simulink model "rpoco8_100_r2"  (R2013a)
settings: Solver=VariableStepDiscrete  SolverMode=SingleTasking  StartTime=0.0  StopTime=10.0  RelTol=1e-3
libraries: xbsIndex_r4 x2263, casper_library_misc x52, casper_library_multipliers x19, xps_library x5, casper_library_sources x4, casper_library_delays x1
(part 1 of 27)
settings Model: Creator=mdexter  LastModifiedBy=domagalski
settings DataIOCC: SignalLoggingSaveFormat=ModelDataLogs
settings OptimizationCC: InlineParams=on  ExpressionDepthLimit=2147483647
settings DebuggingCC: FcnCallInpInsideContextMsg=EnableAllAsWarning

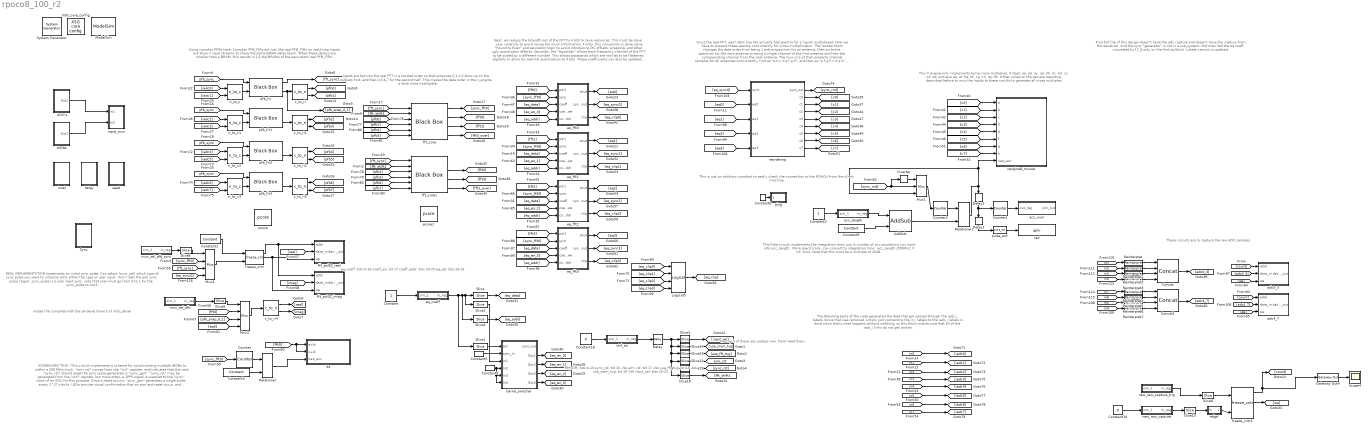
== system rpoco8_100_r2 ==
  note: model file compiled with the s6-devel branch of mlib_devel
  note: !DISREGARD THIS !
      |
      | This circuit implements a scheme for synchronizing
      | multiple IBOBs to within a 200 MHz clock.  "arm_rst"
      | comes from the "ctrl" register, and indicates that the
      | next "sync_rst" should reset the sync pulse generated
      | in "sync_gen".  "sync_rst" may be generated from
      | the "ctrl" register, but more often, a 1PPS signal is
      | supplied to the "sync" input of an ADC for this
      | purpose.  Once a reset occurs, "sync_gen" generates
      | a single pulse every 2^27 clocks.  LEDs provide visual
      | confirmation that an arm and reset occur, and "mrst"
      | is passed over XAUI for the purpose of informing
      | downstream logic in a packetized correlator that
      | a "master reset" has occurred.
  note: Next, we reduce the bitwidth out of the FFT to 4 bits to save resources.
      | This must be done very carefully to avoid losing too much information.
      | Firstly, this conversion is done using "Round to Even" and saturation
      | logic to avoid introducing DC offsets, wrapping, and other ugly quantizaton
      | effects.  Secondly, the "equalizer" allows each frequency channel of the
      | FFT to be scaled by a different number.  This allows passbands which are
      | not flat to be flattened digitally to allow for optimal quantization to 4 bits.
      | These coefficients can also be updated dynamically for gain control.
      | Coefficients can be dynamically written into the "equalizer" by
      | specifying the channel ("coeff_addr") and the value of the
      | coefficient ("coeff"), and then using "coeff_en" to write the
      | new coefficient into the equalization table.
  note: eq_coeff: bits 0-16
      | coeff_en: bit 17
      | coeff_addr: bits 20-25
      | eq_sel: bits 28-31
  note: fft_shift: bits 0-15
      | sync_rst: bit 16 -NA
      | arm_rst: bit 17 -NA
      | use_fft_tvg: bit 18 -NA
      | use_sram_tvg: bit 19 -NA
      | input_sel: bits 20-22
  note: Since the real-FFT, each data line has actually had spectra for 2 inputs multiplexed.
      | Now we have to present these spectra concurrently for cross-multiplication.  The reorder
      | block changes the data order from being 1 entire spectrum for an antenna, then an entire
      | spectrum for the next antenna to being a single channel of the first antenna and then the
      | corresponding channel from the next antenna.  The mux circuit then presents channel
      | samples for all antennas concurrently, first as "a b c d e f g h", and then as "e f g h c d a b".
      | We can post samples twice b/c for 8 data lines, data is only valid 1/2 the time.  By posting
      | samples twice with permuted order, we can cut out some cmults in the xengine that follows.
  note: This X engine only implements some cross-multiplies.  It does:
      | aa, ab, ac, ad, bb, bc, bd, cc, cd, dd, and also
      | ae, af, be, bf, cg, ch, dg, dh.  It then relies on the sample
      | reposting described before to mux the inputs to these
      | cmults to generate all cross multiples.
  note: Inputs are fed into the real FFT in a twisted order
      | so that antennas 0,1,2,3 show up on the outputs first,
      | and then 4,5,6,7 for the second half.  This makes the
      | data order in the x_engine a little more intelligible.
  note: Using complex PFBs here.  Complex PFB_FIRs act just like real
      | PFB_FIRs on real/imag inputs, but  allow 2 input streams to
      | share the same BRAM delay block.  When these delays are smaller
      | than a BRAM, this results in 1/2 the BRAMs of the equivalent real
      | PFB_FIRs.
  note: the top 5 of these are
      | useless now. Dont
      | need them.
  note: REAL IMPLEMENTATION
      |
      | Impements an initial sync pulse.
      | Can select (sync_sel) which type of
      | sync pulse you want to initialize with; either the
      | 1pps or  user input.
      | "Arm"  sets the adc sync pulse (1pps).
      | sync_pulse is a user  input sync. note that
      | user must go from 0 to 1 for the sync_pulse to
      | work.
  note: This little circuit implements the integration time.
      | put in number of accumulations you want into acc_length..
      | More specifically,  can convert to integration time : acc_length /200MHz = int. time.
      | Note that  this must be a multiple of 2048.
  note: These circuits are to capture the raw ADC samples.
  note: First bof file of this design doesn't have the adc
      | capture and doesn't have the capture from the
      | equalizer. And the sync "generator" is not in a sub_system.
      | Old ones had the  eq coeff converted to 17_6 only on the
      | first eq block.
      | Latest version is updated.
  note: The Walshing parts of the code generated the data
      | that got passed through the iadc_i labels. Since that
      | was removed, simply just connecting the in_i labels to
      | the iadc_i labels is done since that's what happens
      | without walshing, so this block makes sure that all of
      | the iadc_i links do not get broken.
  note: This is just an arbitrary constant to
      | easily check the connection to the
      | ROACH from the client machine.
  " System Generator" : xbsIndex_r4/ System Generator  Tag=genX  xilinxfamily=virtex6  part=xc6vsx475t  speed=-1  package=ff1759  synthesis_tool=XST  clock_wrapper=Clock Enables  directory=./rpoco8_r2/sysgen  proj_type=Project Navigator  Synth_file=XST Defaults  Impl_file=ISE Defaults  testbench=off  simulink_period=1  sysclk_period=5  dcm_input_clock_period=100  incr_netlist=off  trim_vbits=Everywhere in SubSystem  dbl_ovrd=According to Block Masks  core_generation=According to Block Masks  run_coregen=off  deprecated_control=off  eval_field=0  block_type=sysgen
      settings: block_version=10.1.3
  ADC's : Subsystem
  AddSub : xbsIndex_r4/AddSub  mode=Subtraction  use_carryin=off  use_carryout=off  en=off  latency=1  precision=Full  arith_type=Unsigned  n_bits=16  bin_pt=14  quantization=Truncate  overflow=Wrap  dbl_ovrd=off  use_behavioral_HDL=off  hw_selection=Fabric  pipelined=off  block_type=addsub
  Concat : xbsIndex_r4/Concat  num_inputs=4  dbl_ovrd=off  block_type=concat
  Concat1 : xbsIndex_r4/Concat  num_inputs=4  dbl_ovrd=off  block_type=concat
  Constant : Constant
  Constant1 : xbsIndex_r4/Constant  const=1  gui_display_data_type=Fixed-point  arith_type=Boolean  n_bits=16  bin_pt=14  preci_type=Single  exp_width=8  frac_width=24  explicit_period=off  period=1  equ=P=C  opselect=C  inp2=PCIN>>17  opr=+  inp1=P  carry=CIN  dbl_ovrd=off  block_type=constant
      settings: block_version=11.4
  Constant10 : Constant  Value=0
  Constant18 : Constant  Value=0
  Constant2 : Constant
  Constant3 : xbsIndex_r4/Constant  const=2^27 - 1  gui_display_data_type=Fixed-point  arith_type=Unsigned  n_bits=27  bin_pt=0  preci_type=Single  exp_width=8  frac_width=24  explicit_period=off  period=1  equ=P=C  opselect=C  inp2=PCIN>>17  opr=+  inp1=P  carry=CIN  dbl_ovrd=off  block_type=constant
      settings: block_version=11.4
  Constant4 : xbsIndex_r4/Constant  const=0  gui_display_data_type=Fixed-point  arith_type=Boolean  n_bits=16  bin_pt=14  preci_type=Single  exp_width=8  frac_width=24  explicit_period=off  period=1  equ=P=C  opselect=C  inp2=PCIN>>17  opr=+  inp1=P  carry=CIN  dbl_ovrd=off  block_type=constant
  Constant5 : xbsIndex_r4/Constant  const=0  gui_display_data_type=Fixed-point  arith_type=Boolean  n_bits=16  bin_pt=14  preci_type=Single  exp_width=8  frac_width=24  explicit_period=on  period=1  equ=P=C  opselect=C  inp2=PCIN>>17  opr=+  inp1=P  carry=CIN  dbl_ovrd=off  block_type=constant
  Constant6 : xbsIndex_r4/Constant  const=1  gui_display_data_type=Fixed-point  arith_type=Unsigned  n_bits=32  bin_pt=0  preci_type=Single  exp_width=8  frac_width=24  explicit_period=off  period=1  equ=P=C  opselect=C  inp2=PCIN>>17  opr=+  inp1=P  carry=CIN  dbl_ovrd=off  block_type=constant
      settings: block_version=11.4
  Constant9 : xbsIndex_r4/Constant  const=1  gui_display_data_type=Fixed-point  arith_type=Unsigned  n_bits=32  bin_pt=0  preci_type=Single  exp_width=8  frac_width=24  explicit_period=off  period=1  equ=P=C  opselect=C  inp2=PCIN>>17  opr=+  inp1=P  carry=CIN  dbl_ovrd=off  block_type=constant
      settings: block_version=11.4
  Counter : xbsIndex_r4/Counter  cnt_type=Free Running  cnt_to=Inf  operation=Up  start_count=0  cnt_by_val=1  arith_type=Unsigned  n_bits=27  bin_pt=0  load_pin=off  rst=on  en=off  explicit_period=on  period=1  dbl_ovrd=off  use_behavioral_HDL=off  implementation=Fabric  block_type=counter
      settings: block_version=11.4
  Counter1 : xbsIndex_r4/Counter  cnt_type=Free Running  cnt_to=Inf  operation=Up  start_count=0  cnt_by_val=1  arith_type=Unsigned  n_bits=32  bin_pt=0  load_pin=off  rst=off  en=on  explicit_period=off  period=1  dbl_ovrd=off  use_behavioral_HDL=off  implementation=Fabric  use_rpm=on  block_type=counter
      settings: xl_area=[0, 0, 0, 0, 0, 0, 0]
  Counter2 : xbsIndex_r4/Counter  cnt_type=Free Running  cnt_to=Inf  operation=Up  start_count=0  cnt_by_val=1  arith_type=Unsigned  n_bits=32  bin_pt=0  load_pin=off  rst=on  en=off  explicit_period=off  period=1  dbl_ovrd=off  use_behavioral_HDL=off  implementation=Fabric  use_rpm=on  block_type=counter
      settings: xl_area=[0, 0, 0, 0, 0, 0, 0]
  Delay : xbsIndex_r4/Delay  rst=off  infoeditControl=Selection of Reset will increase slice count due to use of real FFs and instead of SRLs  en=off  latency=1  dbl_ovrd=off  reg_retiming=off  block_type=delay
  Delay2 : xbsIndex_r4/Delay  rst=off  infoeditControl=Selection of Reset will increase slice count due to use of real FFs and instead of SRLs  en=off  latency=4  dbl_ovrd=off  reg_retiming=on  block_type=delay
      settings: xl_area=[0, 0, 0, 0, 0, 0, 0]
  Delay3 : xbsIndex_r4/Delay  rst=off  infoeditControl=Selection of Reset will increase slice count due to use of real FFs and instead of SRLs  en=off  latency=4  dbl_ovrd=off  reg_retiming=on  block_type=delay
      settings: xl_area=[0, 0, 0, 0, 0, 0, 0]
  Gateway Out4 : xbsIndex_r4/Gateway Out  inherit_from_input=off  hdl_port=on  timing_constraint=None  locs_specified=off  LOCs={}  UseAsDAC=off  DACChannel='1'  block_type=gatewayout
      settings: infoedit="Gateway out block.  Converts Xilinx fixed point inputs into ouputs of type Simulink integer, double, or fixed point.<br><br>Hardware notes:  In hardware these blocks become top level output ports or are discarded, depending on how they are configured."  block_version=11.4
  Inverter : xbsIndex_r4/Inverter  en=off  latency=0  dbl_ovrd=off  block_type=inv
      settings: block_version=11.4
  Logical5 : xbsIndex_r4/Logical  logical_function=OR  inputs=4  en=off  latency=0  precision=Full  arith_type=Unsigned  n_bits=8  bin_pt=2  align_bp=on  dbl_ovrd=off  block_type=logical
      settings: xl_area=[0, 0, 0, 0, 0, 0, 0]
  ModelSim : xbsIndex_r4/ModelSim  dir=./modelsim  waveform=on  leave_open=on  skip_compile=off  use_unisim=off  use_ver_xilinxcorelib=off  custom_scripts=off  startup_timeout=40  block_type=hdlcosim
      settings: infoedit="Allow other blocks to schedule HDL co-simulation tasks.<P><P>Note that selecting \"Skip compilation\" when inappropriate can cause simulation errors and failures. Please refer to the block help for details."  block_version=10.1.3
  Mux1 : xbsIndex_r4/Mux  inputs=2  en=off  latency=0  precision=Full  arith_type=Unsigned  n_bits=16  bin_pt=14  quantization=Truncate  overflow=Wrap  dbl_ovrd=off  block_type=mux
      settings: block_version=11.4
  Mux2 : xbsIndex_r4/Mux  inputs=3  en=off  latency=0  precision=Full  arith_type=Unsigned  n_bits=16  bin_pt=14  quantization=Truncate  overflow=Wrap  dbl_ovrd=off  block_type=mux
      settings: block_version=11.4
  Mux3 : xbsIndex_r4/Mux  inputs=3  en=off  latency=0  precision=Full  arith_type=Unsigned  n_bits=16  bin_pt=14  quantization=Truncate  overflow=Wrap  dbl_ovrd=off  block_type=mux
      settings: block_version=11.4
  Reinterpret{,1..7} (8 alike) : xbsIndex_r4/Reinterpret  force_arith_type=on  arith_type=Unsigned  force_bin_pt=on  bin_pt=0  block_type=reinterpret
      settings: infoedit="Changes signal type without altering the binary representation.   You can changed the signal between signed and unsigned, and relocate the binary point.<br><br>Hardware notes: In hardware this block costs nothing.<br><br>Example:  Suppose the input is 6 bits wide, signed, with 2 fractional bits, and the output is forced to unsigned with 0 fractional bits.  Then an input of -2.0 (1110.00 in binary 2's complement) becomes an output of 56 (111000 in binary)."
  Relational : xbsIndex_r4/Relational  mode=a=b  en=off  latency=0  dbl_ovrd=off  block_type=relational
  Relational1 : xbsIndex_r4/Relational  mode=a=b  en=off  latency=0  dbl_ovrd=off  block_type=relational
  Scope4 : Scope
  Slice : xbsIndex_r4/Slice  nbits=17  boolean_output=off  mode=Lower Bit Location + Width  bit1=0  base1=MSB of Input  bit0=0  base0=LSB of Input  dbl_ovrd=off  block_type=slice
      settings: infoedit="Extracts a given range of bits from each input sample and presents it at the output.  The output type is ordinarily unsigned with binary point at zero, but can be Boolean when the slice is one bit wide.<P><P>Hardware notes: In hardware this block costs nothing."  block_version=10.1.3
  Slice1 : xbsIndex_r4/Slice  nbits=2  boolean_output=off  mode=Lower Bit Location + Width  bit1=0  base1=MSB of Input  bit0=28  base0=LSB of Input  dbl_ovrd=off  block_type=slice
      settings: block_version=10.1.3
  Slice10 : xbsIndex_r4/Slice  nbits=1  boolean_output=on  mode=Lower Bit Location + Width  bit1=0  base1=MSB of Input  bit0=0  base0=LSB of Input  dbl_ovrd=off  block_type=slice
  Slice18 : xbsIndex_r4/Slice  nbits=16  boolean_output=off  mode=Lower Bit Location + Width  bit1=0  base1=MSB of Input  bit0=0  base0=LSB of Input  dbl_ovrd=off  block_type=slice
      settings: block_version=10.1.3
  Slice19 : xbsIndex_r4/Slice  nbits=1  boolean_output=on  mode=Lower Bit Location + Width  bit1=0  base1=MSB of Input  bit0=16  base0=LSB of Input  dbl_ovrd=off  block_type=slice
      settings: infoedit="Extracts a given range of bits from each input sample and presents it at the output.  The output type is ordinarily unsigned with binary point at zero, but can be Boolean when the slice is one bit wide.<P><P>Hardware notes: In hardware this block costs nothing."  block_version=10.1.3
  Slice2 : xbsIndex_r4/Slice  nbits=1  boolean_output=on  mode=Lower Bit Location + Width  bit1=0  base1=MSB of Input  bit0=17  base0=LSB of Input  dbl_ovrd=off  block_type=slice
      settings: block_version=10.1.3
  Slice22 : xbsIndex_r4/Slice  nbits=1  boolean_output=on  mode=Lower Bit Location + Width  bit1=0  base1=MSB of Input  bit0=17  base0=LSB of Input  dbl_ovrd=off  block_type=slice
      settings: infoedit="Extracts a given range of bits from each input sample and presents it at the output.  The output type is ordinarily unsigned with binary point at zero, but can be Boolean when the slice is one bit wide.<P><P>Hardware notes: In hardware this block costs nothing."  block_version=10.1.3
  Slice23 : xbsIndex_r4/Slice  nbits=1  boolean_output=off  mode=Lower Bit Location + Width  bit1=0  base1=MSB of Input  bit0=18  base0=LSB of Input  dbl_ovrd=off  block_type=slice
      settings: infoedit="Extracts a given range of bits from each input sample and presents it at the output.  The output type is ordinarily unsigned with binary point at zero, but can be Boolean when the slice is one bit wide.<P><P>Hardware notes: In hardware this block costs nothing."  block_version=10.1.3
  Slice24 : xbsIndex_r4/Slice  nbits=1  boolean_output=off  mode=Lower Bit Location + Width  bit1=0  base1=MSB of Input  bit0=19  base0=LSB of Input  dbl_ovrd=off  block_type=slice
      settings: infoedit="Extracts a given range of bits from each input sample and presents it at the output.  The output type is ordinarily unsigned with binary point at zero, but can be Boolean when the slice is one bit wide.<P><P>Hardware notes: In hardware this block costs nothing."  block_version=10.1.3
  Slice3 : xbsIndex_r4/Slice  nbits=3  boolean_output=off  mode=Lower Bit Location + Width  bit1=0  base1=MSB of Input  bit0=20  base0=LSB of Input  dbl_ovrd=off  block_type=slice
      settings: infoedit="Extracts a given range of bits from each input sample and presents it at the output.  The output type is ordinarily unsigned with binary point at zero, but can be Boolean when the slice is one bit wide.<P><P>Hardware notes: In hardware this block costs nothing."  block_version=10.1.3
  Slice4 : xbsIndex_r4/Slice  nbits=6  boolean_output=off  mode=Lower Bit Location + Width  bit1=0  base1=MSB of Input  bit0=20  base0=LSB of Input  dbl_ovrd=off  block_type=slice
      settings: block_version=10.1.3
  Slice6 : xbsIndex_r4/Slice  nbits=1  boolean_output=on  mode=Lower Bit Location + Width  bit1=0  base1=MSB of Input  bit0=0  base0=LSB of Input  dbl_ovrd=off  block_type=slice
  Slice8 : xbsIndex_r4/Slice  nbits=2  boolean_output=off  mode=Lower Bit Location + Width  bit1=0  base1=MSB of Input  bit0=0  base0=LSB of Input  dbl_ovrd=off  block_type=slice
  Slice9 : xbsIndex_r4/Slice  nbits=2  boolean_output=off  mode=Lower Bit Location + Width  bit1=0  base1=MSB of Input  bit0=0  base0=LSB of Input  dbl_ovrd=off  block_type=slice
  Sync : Subsystem  mask{reg_latency=2, mux_latency=2}
      mask prompts: reg_latency "Register Latency"; mux_latency "Mux Latency"
  WGNs : Subsystem
  XSG_core_config : xps_library/XSG core config  Tag=xps:xsg  hw_sys=ROACH2:sx475t  clk_src=adc0_clk  ROACH_clk_src=adc0_clk  ROACH2_clk_src=adc0_clk  MKDIG_clk_src=sys_clk  clk_rate=200  sample_period=1  synthesis_tool=XST
  aa : Subsystem
  acc_length : Subsystem  Tag=xps:sw_reg  AncestorBlock=xps_library/software register  mask(swreg){mode=one value, io_dir=From Processor, io_delay=0, sample_period=1, names=reg, bitwidths=32, arith_types=0, bin_pts=0, sim_port=on, show_format=off}
      mask prompts: io_dir "I/O direction"; io_delay "I/O delay"; sample_period "Sample period"; names "Name:"; bitwidths "Bitwidth:"; arith_types "Type (ufix=0, fix=1, bool=2):"; bin_pts "Binary pt:"; sim_port "Provide sim input/output?"; show_format "Print format string?"
      mask init:
      | swreg_init(gcb)
      settings: AttributesFormatString=1input
      mask TypeOptions mode: one value | fields of equal size | fields of arbitrary size
      mask Callback mode: swreg_cb(gcb);
      mask TypeOptions io_dir: To Processor | From Processor
      mask Callback io_dir:
      | mask_enables = get_param(gcb, 'MaskEnables');
      | mask_names = get_param(gcb, 'MaskNames');
      | if strcmp(get_param(gcb, 'io_dir'), 'To Processor'),
      |     mask_enables{ismember(mask_names, 'sample_period')} = 'off';
      | else
      |     mask_enables{ismember(mask_names, 'sample_period')} = 'on';
      | end
      | set_param(gcb, 'MaskEnables', mask_enables);
      mask Callback bitwidths: swreg_maskcheck(gcb);
      mask Callback arith_types: [numios, ~, ~, ~, current_types] = swreg_maskcheck(gcb);
      mask Callback bin_pts: swreg_maskcheck(gcb);
  acc_num : Subsystem  Tag=xps:sw_reg  AncestorBlock=xps_library/software register  mask(swreg){mode=one value, io_dir=To Processor, io_delay=0, sample_period=1, names=reg, bitwidths=32, arith_types=0, bin_pts=0, sim_port=on, show_format=off}
      mask prompts: io_dir "I/O direction"; io_delay "I/O delay"; sample_period "Sample period"; names "Name:"; bitwidths "Bitwidth:"; arith_types "Type (ufix=0, fix=1, bool=2):"; bin_pts "Binary pt:"; sim_port "Provide sim input/output?"; show_format "Print format string?"
      mask init:
      | swreg_init(gcb)
      settings: AttributesFormatString=1output
      mask TypeOptions mode: one value | fields of equal size | fields of arbitrary size
      mask Callback mode: swreg_cb(gcb);
      mask TypeOptions io_dir: To Processor | From Processor
      mask Callback io_dir:
      | mask_enables = get_param(gcb, 'MaskEnables');
      | mask_names = get_param(gcb, 'MaskNames');
      | if strcmp(get_param(gcb, 'io_dir'), 'To Processor'),
      |     mask_enables{ismember(mask_names, 'sample_period')} = 'off';
      | else
      |     mask_enables{ismember(mask_names, 'sample_period')} = 'on';
      | end
      | set_param(gcb, 'MaskEnables', mask_enables);
      mask Callback bitwidths: swreg_maskcheck(gcb);
      mask Callback arith_types: [numios, ~, ~, ~, current_types] = swreg_maskcheck(gcb);
      mask Callback bin_pts: swreg_maskcheck(gcb);
  adc0_3 : Subsystem  Tag=xps:bram  AncestorBlock=xps_library/Shared BRAM  mask{arith_type=Unsigned, addr_width=11, data_width=32, reg_prim_output=off, reg_core_output=off, optimization=Minimum_Area, data_bin_pt=0, init_vals=[1:2^10-1], sample_rate=1}
      mask prompts: arith_type "Output Data Type"; addr_width "Address width"; data_width "Data Width"; reg_prim_output "Register Primitive Output"; reg_core_output "Register Core Output"; data_bin_pt "Data Binary Point"; init_vals "Initial values (simulation only)"; sample_rate "Sample rate"
      mask init:
      | shared_bram_mask;
      mask TypeOptions arith_type: Unsigned | Signed  (2's comp)
      mask TypeOptions data_width: 8 | 16 | 32 | 64 | 128
      mask TypeOptions optimization: Minimum_Area | Low_Power
  adc4_7 : Subsystem  Tag=xps:bram  AncestorBlock=xps_library/Shared BRAM  mask{arith_type=Unsigned, addr_width=11, data_width=32, reg_prim_output=off, reg_core_output=off, optimization=Minimum_Area, data_bin_pt=0, init_vals=[1:2^10-1], sample_rate=1}
      mask prompts: arith_type "Output Data Type"; addr_width "Address width"; data_width "Data Width"; reg_prim_output "Register Primitive Output"; reg_core_output "Register Core Output"; data_bin_pt "Data Binary Point"; init_vals "Initial values (simulation only)"; sample_rate "Sample rate"
      mask init:
      | shared_bram_mask;
      mask TypeOptions arith_type: Unsigned | Signed  (2's comp)
      mask TypeOptions data_width: 8 | 16 | 32 | 64 | 128
      mask TypeOptions optimization: Minimum_Area | Low_Power
  barrel_switcher : Subsystem  AncestorBlock=casper_library_reorder/barrel_switcher  mask(barrel_switcher){n_inputs=2, async=off}
      mask prompts: n_inputs "Number of Inputs: (2^?)"; async "Asynchronous operation"
      mask help:
      | Shifts input to right by amount specified on sel,
      | wrapping around into higher order bits.
      mask init:
      | barrel_switcher_init(gcb,...
      |     'n_inputs', n_inputs, ...
      |     'async', async);
      mask Help: eval('xlWeb(''http://casper.berkeley.edu/wiki/Barrel_switcher'')')
  c_to_ri{,1..4} (5 alike) : casper_library_misc/c_to_ri  n_bits=18  bin_pt=17
  ctrl_sw : Subsystem  Tag=xps:sw_reg  AncestorBlock=xps_library/software register  mask(swreg){mode=one value, io_dir=From Processor, io_delay=0, sample_period=1, names=reg, bitwidths=32, arith_types=0, bin_pts=0, sim_port=on, show_format=off}
      mask prompts: io_dir "I/O direction"; io_delay "I/O delay"; sample_period "Sample period"; names "Name:"; bitwidths "Bitwidth:"; arith_types "Type (ufix=0, fix=1, bool=2):"; bin_pts "Binary pt:"; sim_port "Provide sim input/output?"; show_format "Print format string?"
      mask init:
      | swreg_init(gcb)
      settings: AttributesFormatString=1input
      mask TypeOptions mode: one value | fields of equal size | fields of arbitrary size
      mask Callback mode: swreg_cb(gcb);
      mask TypeOptions io_dir: To Processor | From Processor
      mask Callback io_dir:
      | mask_enables = get_param(gcb, 'MaskEnables');
      | mask_names = get_param(gcb, 'MaskNames');
      | if strcmp(get_param(gcb, 'io_dir'), 'To Processor'),
      |     mask_enables{ismember(mask_names, 'sample_period')} = 'off';
      | else
      |     mask_enables{ismember(mask_names, 'sample_period')} = 'on';
      | end
      | set_param(gcb, 'MaskEnables', mask_enables);
      mask Callback bitwidths: swreg_maskcheck(gcb);
      mask Callback arith_types: [numios, ~, ~, ~, current_types] = swreg_maskcheck(gcb);
      mask Callback bin_pts: swreg_maskcheck(gcb);
  delay : Subsystem  mask{addr_offset=8195}
      mask prompts: addr_offset "Address"
      mask init:
      | start_addr = (addr_offset);
      | fmtstr = sprintf('Addr %d\n0x%04X', start_addr, start_addr);
      | set_param(gcb, 'AttributesFormatString', fmtstr);
      settings: AttributesFormatString=|
      | Addr 8195
      | 0x2003
  edge : Subsystem  AncestorBlock=casper_library_misc/edge_detect  mask(edge_detect){edge=Both, polarity=Active High, x_in=[0 0.08 0.08 0.16 0.16 0.24 0.24 0.32 0.32 0.4], y_in=[-1 -1  1  1  1  1  1  1  1  1], x_out=[0.6 0.68 0.68 0.76 0.76 0.84 0.84 0.92 0.92 1], y_out=[-1 -1  1  1 -1 -1 -1 -1 -1 -1]}
      mask prompts: edge "Edge Type"; polarity "Output Polarity"; x_in "Input X Positions"; y_in "Input Y Positions"; x_out "Output X Positions"; y_out "Output Y Positions"
      mask help: Output is active for one-cycle after each edge of the specified type (i.e. rising, falling or both).
      mask init:
      | edge_detect_init(gcb,...
      |     'edge',edge,...
      |     'polarity',polarity,...
      |     'x_in',x_in,...
      |     'x_out',x_out,...
      |     'y_in',y_in,...
      |     'y_out',y_out);
      | 
      | x_in_num=str2num(getfield(getfield(get_param(gcb,'UserData'),'parameters'),'x_in'));
      | x_out_num=str2num(getfield(getfield(get_param(gcb,'UserData'),'parameters'),'x_out'));
      | y_in_num=str2num(getfield(getfield(get_param(gcb,'UserData'),'parameters'),'y_in'));
      | y_out_num=str2num(getfield(getfield(get_param(gcb,'UserData'),'parameters'),'y_out'));
      settings: AttributesFormatString=|
      | both edges
      | active high
      mask Help: Output is active for one-cycle after each edge of the specified type (i.e. rising, falling, or both).  Latency is zero.
      mask TypeOptions edge: Rising | Falling | Both
      mask TypeOptions polarity: Active High | Active Low
      mask Display:
      | plot(x_in_num,0.5+y_in_num*0.2);
      | plot(x_out_num,0.5+y_out_num*0.2);
  eq_coeff : Subsystem  Tag=xps:sw_reg  AncestorBlock=xps_library/software register  mask(swreg){mode=one value, io_dir=From Processor, io_delay=0, sample_period=1, names=reg, bitwidths=32, arith_types=0, bin_pts=0, sim_port=on, show_format=off}
      mask prompts: io_dir "I/O direction"; io_delay "I/O delay"; sample_period "Sample period"; names "Name:"; bitwidths "Bitwidth:"; arith_types "Type (ufix=0, fix=1, bool=2):"; bin_pts "Binary pt:"; sim_port "Provide sim input/output?"; show_format "Print format string?"
      mask init:
      | swreg_init(gcb)
      settings: AttributesFormatString=1input
      mask TypeOptions mode: one value | fields of equal size | fields of arbitrary size
      mask Callback mode: swreg_cb(gcb);
      mask TypeOptions io_dir: To Processor | From Processor
      mask Callback io_dir:
      | mask_enables = get_param(gcb, 'MaskEnables');
      | mask_names = get_param(gcb, 'MaskNames');
      | if strcmp(get_param(gcb, 'io_dir'), 'To Processor'),
      |     mask_enables{ismember(mask_names, 'sample_period')} = 'off';
      | else
      |     mask_enables{ismember(mask_names, 'sample_period')} = 'on';
      | end
      | set_param(gcb, 'MaskEnables', mask_enables);
      mask Callback bitwidths: swreg_maskcheck(gcb);
      mask Callback arith_types: [numios, ~, ~, ~, current_types] = swreg_maskcheck(gcb);
      mask Callback bin_pts: swreg_maskcheck(gcb);
  eq_fft0 : Subsystem  mask{nchan=11}
      mask prompts: nchan "FFT Channels (2^?):"
  eq_fft1 : Subsystem  mask{nchan=11}
      mask prompts: nchan "FFT Channels (2^?):"
  eq_fft2 : Subsystem  mask{nchan=11}
      mask prompts: nchan "FFT Channels (2^?):"
  eq_fft3 : Subsystem  mask{nchan=11}
      mask prompts: nchan "FFT Channels (2^?):"
  fft_core : xbsIndex_r4/Black Box  init_code=fft_core_v6_config  sim_method=Inactive  verbose=off  block_type=blackbox2
  fft_core1 : xbsIndex_r4/Black Box  init_code=fft_core_v6_config  sim_method=Inactive  verbose=off  block_type=blackbox2
  fft_pol02_imag : Subsystem  Tag=xps:bram  AncestorBlock=xps_library/Shared BRAM  mask{arith_type=Unsigned, addr_width=11, data_width=32, reg_prim_output=off, reg_core_output=off, optimization=Minimum_Area, data_bin_pt=0, init_vals=[1:2^10-1], sample_rate=1}
      mask prompts: arith_type "Output Data Type"; addr_width "Address width"; data_width "Data Width"; reg_prim_output "Register Primitive Output"; reg_core_output "Register Core Output"; data_bin_pt "Data Binary Point"; init_vals "Initial values (simulation only)"; sample_rate "Sample rate"
      mask init:
      | shared_bram_mask;
      mask TypeOptions arith_type: Unsigned | Signed  (2's comp)
      mask TypeOptions data_width: 8 | 16 | 32 | 64 | 128
      mask TypeOptions optimization: Minimum_Area | Low_Power
  fft_pol02_real : Subsystem  Tag=xps:bram  AncestorBlock=xps_library/Shared BRAM  mask{arith_type=Unsigned, addr_width=11, data_width=32, reg_prim_output=off, reg_core_output=off, optimization=Minimum_Area, data_bin_pt=0, init_vals=[1:2^10-1], sample_rate=1}
      mask prompts: arith_type "Output Data Type"; addr_width "Address width"; data_width "Data Width"; reg_prim_output "Register Primitive Output"; reg_core_output "Register Core Output"; data_bin_pt "Data Binary Point"; init_vals "Initial values (simulation only)"; sample_rate "Sample rate"
      mask init:
      | shared_bram_mask;
      mask TypeOptions arith_type: Unsigned | Signed  (2's comp)
      mask TypeOptions data_width: 8 | 16 | 32 | 64 | 128
      mask TypeOptions optimization: Minimum_Area | Low_Power
  freeze_cntr : casper_library_misc/freeze_cntr  CounterBits=11
  freeze_cntr1 : casper_library_misc/freeze_cntr  CounterBits=11
  input_mux : Subsystem
  insel : Subsystem  mask{addr_offset=8194}
      mask prompts: addr_offset "Address"
      mask init:
      | start_addr = (addr_offset);
      | fmtstr = sprintf('Addr %d\n0x%04X', start_addr, start_addr);
      | set_param(gcb, 'AttributesFormatString', fmtstr);
      settings: AttributesFormatString=|
      | Addr 8194
      | 0x2002
  led : xps_library/gpio  Tag=xps:gpio  io_group=ROACH2:led  io_dir=out  arith_type=Boolean  bitwidth=1  bin_pt=0  bit_index=0  sample_period=1  use_single_ended=off  use_ddr=off  reg_iob=on  reg_clk_phase=0  termination=None
  mux_sel_pfb : Subsystem  Tag=xps:sw_reg  AncestorBlock=xps_library/software register  mask(swreg){mode=one value, io_dir=From Processor, io_delay=0, sample_period=1, names=reg, bitwidths=32, arith_types=0, bin_pts=0, sim_port=on, show_format=off}
      mask prompts: io_dir "I/O direction"; io_delay "I/O delay"; sample_period "Sample period"; names "Name:"; bitwidths "Bitwidth:"; arith_types "Type (ufix=0, fix=1, bool=2):"; bin_pts "Binary pt:"; sim_port "Provide sim input/output?"; show_format "Print format string?"
      mask init:
      | swreg_init(gcb)
      settings: AttributesFormatString=1input
      mask TypeOptions mode: one value | fields of equal size | fields of arbitrary size
      mask Callback mode: swreg_cb(gcb);
      mask TypeOptions io_dir: To Processor | From Processor
      mask Callback io_dir:
      | mask_enables = get_param(gcb, 'MaskEnables');
      | mask_names = get_param(gcb, 'MaskNames');
      | if strcmp(get_param(gcb, 'io_dir'), 'To Processor'),
      |     mask_enables{ismember(mask_names, 'sample_period')} = 'off';
      | else
      |     mask_enables{ismember(mask_names, 'sample_period')} = 'on';
      | end
      | set_param(gcb, 'MaskEnables', mask_enables);
      mask Callback bitwidths: swreg_maskcheck(gcb);
      mask Callback arith_types: [numios, ~, ~, ~, current_types] = swreg_maskcheck(gcb);
      mask Callback bin_pts: swreg_maskcheck(gcb);
  mux_sel_pfb_sync : Subsystem  Tag=xps:sw_reg  AncestorBlock=xps_library/software register  mask(swreg){mode=one value, io_dir=From Processor, io_delay=0, sample_period=1, names=reg, bitwidths=32, arith_types=0, bin_pts=0, sim_port=on, show_format=off}
      mask prompts: io_dir "I/O direction"; io_delay "I/O delay"; sample_period "Sample period"; names "Name:"; bitwidths "Bitwidth:"; arith_types "Type (ufix=0, fix=1, bool=2):"; bin_pts "Binary pt:"; sim_port "Provide sim input/output?"; show_format "Print format string?"
      mask init:
      | swreg_init(gcb)
      settings: AttributesFormatString=1input
      mask TypeOptions mode: one value | fields of equal size | fields of arbitrary size
      mask Callback mode: swreg_cb(gcb);
      mask TypeOptions io_dir: To Processor | From Processor
      mask Callback io_dir:
      | mask_enables = get_param(gcb, 'MaskEnables');
      | mask_names = get_param(gcb, 'MaskNames');
      | if strcmp(get_param(gcb, 'io_dir'), 'To Processor'),
      |     mask_enables{ismember(mask_names, 'sample_period')} = 'off';
      | else
      |     mask_enables{ismember(mask_names, 'sample_period')} = 'on';
      | end
      | set_param(gcb, 'MaskEnables', mask_enables);
      mask Callback bitwidths: swreg_maskcheck(gcb);
      mask Callback arith_types: [numios, ~, ~, ~, current_types] = swreg_maskcheck(gcb);
      mask Callback bin_pts: swreg_maskcheck(gcb);
  new_raw_capture : Subsystem  Tag=xps:sw_reg  AncestorBlock=xps_library/software register  mask(swreg){mode=one value, io_dir=From Processor, io_delay=0, sample_period=1, names=reg, bitwidths=32, arith_types=0, bin_pts=0, sim_port=on, show_format=off}
      mask prompts: io_dir "I/O direction"; io_delay "I/O delay"; sample_period "Sample period"; names "Name:"; bitwidths "Bitwidth:"; arith_types "Type (ufix=0, fix=1, bool=2):"; bin_pts "Binary pt:"; sim_port "Provide sim input/output?"; show_format "Print format string?"
      mask init:
      | swreg_init(gcb)
      settings: AttributesFormatString=1input
      mask TypeOptions mode: one value | fields of equal size | fields of arbitrary size
      mask Callback mode: swreg_cb(gcb);
      mask TypeOptions io_dir: To Processor | From Processor
      mask Callback io_dir:
      | mask_enables = get_param(gcb, 'MaskEnables');
      | mask_names = get_param(gcb, 'MaskNames');
      | if strcmp(get_param(gcb, 'io_dir'), 'To Processor'),
      |     mask_enables{ismember(mask_names, 'sample_period')} = 'off';
      | else
      |     mask_enables{ismember(mask_names, 'sample_period')} = 'on';
      | end
      | set_param(gcb, 'MaskEnables', mask_enables);
      mask Callback bitwidths: swreg_maskcheck(gcb);
      mask Callback arith_types: [numios, ~, ~, ~, current_types] = swreg_maskcheck(gcb);
      mask Callback bin_pts: swreg_maskcheck(gcb);
  new_raw_capture_trig : Subsystem  Tag=xps:sw_reg  AncestorBlock=xps_library/software register  mask(swreg){mode=one value, io_dir=From Processor, io_delay=0, sample_period=1, names=reg, bitwidths=32, arith_types=0, bin_pts=0, sim_port=on, show_format=off}
      mask prompts: io_dir "I/O direction"; io_delay "I/O delay"; sample_period "Sample period"; names "Name:"; bitwidths "Bitwidth:"; arith_types "Type (ufix=0, fix=1, bool=2):"; bin_pts "Binary pt:"; sim_port "Provide sim input/output?"; show_format "Print format string?"
      mask init:
      | swreg_init(gcb)
      settings: AttributesFormatString=1input
      mask TypeOptions mode: one value | fields of equal size | fields of arbitrary size
      mask Callback mode: swreg_cb(gcb);
      mask TypeOptions io_dir: To Processor | From Processor
      mask Callback io_dir:
      | mask_enables = get_param(gcb, 'MaskEnables');
      | mask_names = get_param(gcb, 'MaskNames');
      | if strcmp(get_param(gcb, 'io_dir'), 'To Processor'),
      |     mask_enables{ismember(mask_names, 'sample_period')} = 'off';
      | else
      |     mask_enables{ismember(mask_names, 'sample_period')} = 'on';
      | end
      | set_param(gcb, 'MaskEnables', mask_enables);
      mask Callback bitwidths: swreg_maskcheck(gcb);
      mask Callback arith_types: [numios, ~, ~, ~, current_types] = swreg_maskcheck(gcb);
      mask Callback bin_pts: swreg_maskcheck(gcb);
  pcore : xps_library/pcore  Tag=xps:pcore  pcore_path=pfb_core_v6/pfb_core_v6.ngc
  pcore1 : xps_library/pcore  Tag=xps:pcore  pcore_path=fft_core_v6/fft_core_v6.ngc
  pfb_fir{,1..3} (4 alike) : xbsIndex_r4/Black Box  init_code=pfb_core_v6_config  sim_method=Inactive  verbose=off  block_type=blackbox2
  ping : Subsystem  Tag=xps:sw_reg  AncestorBlock=xps_library/software register  mask(swreg){mode=one value, io_dir=To Processor, io_delay=0, sample_period=1, names=reg, bitwidths=32, arith_types=0, bin_pts=0, sim_port=off, show_format=off}
      mask prompts: io_dir "I/O direction"; io_delay "I/O delay"; sample_period "Sample period"; names "Name:"; bitwidths "Bitwidth:"; arith_types "Type (ufix=0, fix=1, bool=2):"; bin_pts "Binary pt:"; sim_port "Provide sim input/output?"; show_format "Print format string?"
      mask init:
      | swreg_init(gcb)
      settings: AttributesFormatString=1output
      mask TypeOptions mode: one value | fields of equal size | fields of arbitrary size
      mask Callback mode: swreg_cb(gcb);
      mask TypeOptions io_dir: To Processor | From Processor
      mask Callback io_dir:
      | mask_enables = get_param(gcb, 'MaskEnables');
      | mask_names = get_param(gcb, 'MaskNames');
      | if strcmp(get_param(gcb, 'io_dir'), 'To Processor'),
      |     mask_enables{ismember(mask_names, 'sample_period')} = 'off';
      | else
      |     mask_enables{ismember(mask_names, 'sample_period')} = 'on';
      | end
      | set_param(gcb, 'MaskEnables', mask_enables);
      mask Callback bitwidths: swreg_maskcheck(gcb);
      mask Callback arith_types: [numios, ~, ~, ~, current_types] = swreg_maskcheck(gcb);
      mask Callback bin_pts: swreg_maskcheck(gcb);
  pulse_ext : casper_library_misc/pulse_ext  pulse_len=2^22
  reordering : Subsystem  mask{n_bits=18}
      mask prompts: n_bits "Bit Width"
  ri_to_c{,1..3} (4 alike) : casper_library_misc/ri_to_c
  seed : Subsystem  mask{addr_offset=8196}
      mask prompts: addr_offset "Address"
      mask init:
      | start_addr = (addr_offset);
      | fmtstr = sprintf('Addr %d\n0x%04X', start_addr, start_addr);
      | set_param(gcb, 'AttributesFormatString', fmtstr);
      settings: AttributesFormatString=|
      | Addr 8196
      | 0x2004
  xengine8_muxed : Subsystem  mask{mult_latency=3, add_latency=2, nchan=10, n_bits=18}
      mask prompts: mult_latency "Mult Latency"; add_latency "Add Latency"; nchan "Number of Channels per Ant (2^?):"; n_bits "Bit Width"
  tag scope: arm_rst=global
  wires:
  pfb_fir/1 -> [fft_sync]
  Logical5/1 -> [eq_clip]
  [eq_clip0] -> Logical5/1
  [eq_clip1] -> Logical5/2
  [eq_clip2] -> Logical5/3
  [eq_clip3] -> Logical5/4
  eq_coeff/1(in_reg) -> Slice/1, Slice2/1, Slice4/1, Slice1/1
  Constant/1 -> eq_coeff/1(sim_1)
  Slice/1 -> [eq_data]
  Slice4/1 -> [eq_addr]
  Slice18/1 -> [fft_shift]
  Delay/1 -> Slice24/1, Slice23/1, Slice22/1, Slice19/1, Slice18/1, Slice3/1
  ctrl_sw/1(in_reg) -> Delay/1
  Counter1/1 -> acc_num/1(out_reg)
  Delay3/1 -> Counter1/1, Delay2/1
  Relational1/1 -> Delay3/1, xengine8_muxed/9(new_acc), Mux1/3
  [c0] -> xengine8_muxed/1(a)
  [c1] -> xengine8_muxed/2(b)
  [c2] -> xengine8_muxed/3(c)
  [c3] -> xengine8_muxed/4(d)
  [c4] -> xengine8_muxed/5(e)
  [c5] -> xengine8_muxed/6(f)
  [c6] -> xengine8_muxed/7(g)
  [c7] -> xengine8_muxed/8(h)
  [eq0] -> reordering/2(eq0)
  [eq1] -> reordering/3(eq1)
  [eq2] -> reordering/4(eq2)
  [eq3] -> reordering/5(eq3)
  [eq_sync0] -> reordering/1(sync)
  reordering/1(sync_out) -> [sync_rnd]
  reordering/2(c0) -> [c0]
  reordering/3(c1) -> [c1]
  reordering/4(c2) -> [c2]
  reordering/5(c3) -> [c3]
  reordering/6(c4) -> [c4]
  reordering/7(c5) -> [c5]
  reordering/8(c6) -> [c6]
  reordering/9(c7) -> [c7]
  barrel_switcher/2(Out1) -> [eq_en_0]
  barrel_switcher/3(Out2) -> [eq_en_1]
  barrel_switcher/4(Out3) -> [eq_en_2]
  barrel_switcher/5(Out4) -> [eq_en_3]
  Slice2/1 -> barrel_switcher/3(In1)
  Slice1/1 -> barrel_switcher/1(sel)
  Constant4/1 -> barrel_switcher/4(In2), barrel_switcher/6(In4), barrel_switcher/5(In3)
  Constant5/1 -> barrel_switcher/2(sync_in)
  Delay2/1 -> pulse_ext/1
  [iadc0] -> ri_to_c/1
  [iadc1] -> ri_to_c/2
  pfb_fir/2 -> c_to_ri/1, [pfb_snap_0_1]
  c_to_ri/1 -> [pfb0]
  c_to_ri/2 -> [pfb1]
  [pfb_sync] -> pfb_fir1/1
  ri_to_c1/1 -> pfb_fir1/2
  pfb_fir1/2 -> c_to_ri1/1
  [pfb_sync] -> pfb_fir2/1
  ri_to_c2/1 -> pfb_fir2/2
  pfb_fir2/2 -> c_to_ri2/1
  [pfb_sync] -> pfb_fir3/1
  ri_to_c3/1 -> pfb_fir3/2
  pfb_fir3/2 -> c_to_ri3/1
  [iadc2] -> ri_to_c1/1
  [iadc3] -> ri_to_c1/2
  [iadc4] -> ri_to_c2/1
  [iadc5] -> ri_to_c2/2
  [iadc6] -> ri_to_c3/1
  [iadc7] -> ri_to_c3/2
  c_to_ri1/1 -> [pfb2]
  c_to_ri1/2 -> [pfb3]
  c_to_ri2/1 -> [pfb4]
  c_to_ri2/2 -> [pfb5]
  c_to_ri3/1 -> [pfb6]
  c_to_ri3/2 -> [pfb7]
  [fft_sync] -> fft_core/1
  [fft_shift] -> fft_core/2
  [pfb0] -> fft_core/3
  [pfb1] -> fft_core/4
  [pfb4] -> fft_core/5
  [pfb5] -> fft_core/6
  [fft_sync] -> fft_core1/1
  [fft_shift] -> fft_core1/2
  [pfb2] -> fft_core1/3
  [pfb3] -> fft_core1/4
  [pfb6] -> fft_core1/5
  [pfb7] -> fft_core1/6
  fft_core/1 -> [sync_fft0]
  fft_core/2 -> [fft0]
  fft_core/3 -> [fft1]
  fft_core/4 -> [fft0_over]
  fft_core1/2 -> [fft2]
  fft_core1/3 -> [fft3]
  fft_core1/4 -> [fft1_over]
  WGNs/1(Out1) -> input_mux/2(In2)
  ADC's/1(Out1) -> input_mux/1(In1)
  freeze_cntr/1 -> fft_pol02_real/1(addr), fft_pol02_imag/1(addr)
  freeze_cntr/2 -> fft_pol02_real/3(we), fft_pol02_imag/3(we)
  Constant1/1 -> freeze_cntr/1
  c_to_ri4/1 -> [real]
  c_to_ri4/2 -> [imag]
  [real] -> fft_pol02_real/2(data_in)
  [imag] -> fft_pol02_imag/2(data_in)
  [fft0] -> aa/1(a+bi), aa/2(c+di)
  [sync_fft0] -> Counter/1
  Counter/1 -> Relational/1
  Constant3/1 -> Relational/2
  Relational/1 -> aa/3(new_acc)
  Counter2/1 -> Relational1/1
  Constant9/1 -> AddSub/2
  AddSub/1 -> Relational1/2
  [sync_rnd] -> Mux1/2, Inverter/1
  Inverter/1 -> Mux1/1
  Mux1/1 -> Counter2/1
  Constant2/1 -> acc_length/1(sim_1)
  [sync_fft0] -> Mux3/2
  [fft_sync] -> Mux3/3
  mux_sel_pfb_sync/1(in_reg) -> Slice8/1
  [fft0] -> Mux2/2
  [pfb_snap_0_1] -> Mux2/3
  Mux3/1 -> freeze_cntr/2
  Mux2/1 -> c_to_ri4/1
  eq_fft0/1(dout) -> [eq0]
  eq_fft0/2(sync_out) -> [eq_sync0]
  [fft0] -> eq_fft0/1(pol1)
  [eq_data] -> eq_fft0/3(coeff)
  [eq_en_0] -> eq_fft0/4(coeff_we)
  eq_fft0/3(clip) -> [eq_clip0]
  [sync_fft0] -> eq_fft0/2(sync)
  [eq_addr] -> eq_fft0/5(coeff_addr)
  [fft1] -> eq_fft1/1(pol1)
  [sync_fft0] -> eq_fft1/2(sync)
  [eq_data] -> eq_fft1/3(coeff)
  [eq_en_1] -> eq_fft1/4(coeff_we)
  [eq_addr] -> eq_fft1/5(coeff_addr)
  [fft2] -> eq_fft2/1(pol1)
  [sync_fft0] -> eq_fft2/2(sync)
  [eq_data] -> eq_fft2/3(coeff)
  [eq_en_2] -> eq_fft2/4(coeff_we)
  [eq_addr] -> eq_fft2/5(coeff_addr)
  [fft3] -> eq_fft3/1(pol1)
  [sync_fft0] -> eq_fft3/2(sync)
  [eq_data] -> eq_fft3/3(coeff)
  [eq_en_3] -> eq_fft3/4(coeff_we)
  [eq_addr] -> eq_fft3/5(coeff_addr)
  eq_fft1/1(dout) -> [eq1]
  eq_fft1/2(sync_out) -> [eq_sync1]
  eq_fft1/3(clip) -> [eq_clip1]
  eq_fft2/1(dout) -> [eq2]
  eq_fft2/2(sync_out) -> [eq_sync2]
  eq_fft2/3(clip) -> [eq_clip2]
  eq_fft3/1(dout) -> [eq3]
  eq_fft3/2(sync_out) -> [eq_sync3]
  eq_fft3/3(clip) -> [eq_clip3]
  Slice9/1 -> Mux2/1
  Slice8/1 -> Mux3/1
  new_raw_capture/1(in_reg) -> Slice10/1
  freeze_cntr1/1 -> [count], Gateway Out4/1
  Slice10/1 -> edge/1(in)
  freeze_cntr1/2 -> [we]
  edge/1(out) -> freeze_cntr1/2
  Gateway Out4/1 -> Scope4/1
  [count] -> adc0_3/1(addr)
  [we] -> adc0_3/3(we)
  [adc0_3] -> adc0_3/2(data_in)
  Reinterpret/1 -> Concat/1
  Reinterpret1/1 -> Concat/2
  Reinterpret2/1 -> Concat/3
  Reinterpret3/1 -> Concat/4
  Reinterpret4/1 -> Concat1/1
  Reinterpret5/1 -> Concat1/2
  Reinterpret6/1 -> Concat1/3
  Reinterpret7/1 -> Concat1/4
  [in3] -> Reinterpret/1
  [in2] -> Reinterpret1/1
  [in1] -> Reinterpret2/1
  [in0] -> Reinterpret3/1
  [in7] -> Reinterpret4/1
  [in6] -> Reinterpret5/1
  [in5] -> Reinterpret6/1
  [in4] -> Reinterpret7/1
  Concat/1 -> [adc0_3]
  Concat1/1 -> [adc4_7]
  [eq0] -> Mux2/4
  [eq_sync0] -> Mux3/4
  new_raw_capture_trig/1(in_reg) -> Slice6/1
  Slice6/1 -> freeze_cntr1/1
  mux_sel_pfb/1(in_reg) -> Slice9/1
  Constant18/1 -> ctrl_sw/1(sim_1)
  acc_length/1(in_reg) -> AddSub/1
  Constant10/1 -> new_raw_capture/1(sim_1)
  [count] -> adc4_7/1(addr)
  [adc4_7] -> adc4_7/2(data_in)
  [we] -> adc4_7/3(we)
  pulse_ext/1 -> led/1
  [in0] -> [iadc0]
  [in1] -> [iadc1]
  [in2] -> [iadc2]
  [in3] -> [iadc3]
  [in4] -> [iadc4]
  [in5] -> [iadc5]
  [in6] -> [iadc6]
  [in7] -> [iadc7]
  Slice24/1 -> [use_sram_tvg]
  Slice23/1 -> [use_fft_tvg]
  Slice22/1 -> [arm_rst]
  Slice19/1 -> [sync_rst]
  Slice3/1 -> [input_sel]
  [pfb_sync] -> pfb_fir/1
  ri_to_c/1 -> pfb_fir/2
  Constant6/1 -> ping/1(out_reg)

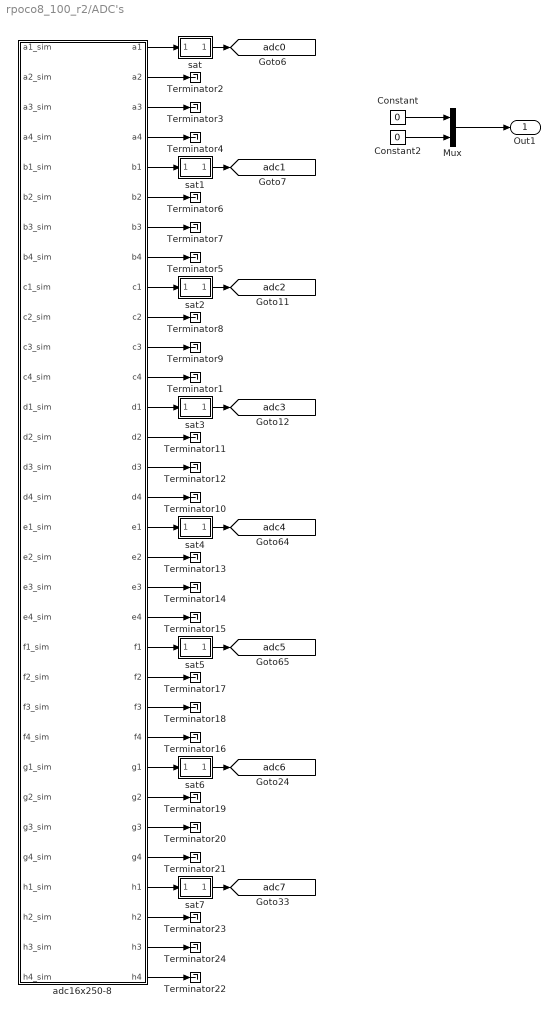
== system rpoco8_100_r2/ADC's ==
  Constant : Constant  Value=0
  Constant2 : Constant  Value=0
  Mux : Mux  Inputs=2
  Terminator{1..24} (24 alike) : Terminator
  adc16x250-8 : Subsystem  Tag=xps:adc16  AncestorBlock=xps_library/ADCs/adc16x250-8  mask(ADC16){board_count=2, roach2_rev=2, zdok_rev=2}
      mask prompts: board_count "Number of ADC16 Boards"; roach2_rev "ROACH2 Revision"; zdok_rev "ZDOK Pinout Revision"
      mask help: 16-input ADC. When using one ADC16 board, it must be in ZDOK0.
      mask init:
      | % Only board_count is needed by init function
      | adc16_init(gcb, ...
      |     'board_count', board_count);
      settings: AttributesFormatString=r2 rev%<roach2_rev>\nzdok rev%<zdok_rev>
      mask Help:
      | This is the CASPER "yellow block" for the CASPER ADC16 board.  Each ADC
      | board has four ADC chips.  Each ADC chip accepts four inputs.  The four
      | 8-bit outputs from each ADC chip are concatenated into a 32-bit signal.
      mask TypeOptions board_count: 1 | 2
      mask TypeOptions roach2_rev: 1 | 2
      mask TypeOptions zdok_rev: 1 | 2
  sat : Subsystem
  sat1 : Subsystem
  sat2 : Subsystem
  sat3 : Subsystem
  sat4 : Subsystem
  sat5 : Subsystem
  sat6 : Subsystem
  sat7 : Subsystem
  Out1 : Outport
  tag scope: adc0=global, adc1=global, adc2=global, adc3=global, adc4=global, adc5=global, adc6=global, adc7=global
  wires:
  sat/1(Out1) -> [adc0]
  sat1/1(Out1) -> [adc1]
  sat2/1(Out1) -> [adc2]
  sat3/1(Out1) -> [adc3]
  sat4/1(Out1) -> [adc4]
  sat5/1(Out1) -> [adc5]
  sat6/1(Out1) -> [adc6]
  sat7/1(Out1) -> [adc7]
  Mux/1 -> Out1/1
  Constant/1 -> Mux/1
  Constant2/1 -> Mux/2
  adc16x250-8/1(a1) -> sat/1(In2)
  adc16x250-8/2(a2) -> Terminator2/1
  adc16x250-8/3(a3) -> Terminator3/1
  adc16x250-8/4(a4) -> Terminator4/1
  adc16x250-8/6(b2) -> Terminator6/1
  adc16x250-8/7(b3) -> Terminator7/1
  adc16x250-8/9(c1) -> sat2/1(In2)
  adc16x250-8/10(c2) -> Terminator8/1
  adc16x250-8/11(c3) -> Terminator9/1
  adc16x250-8/12(c4) -> Terminator1/1
  adc16x250-8/14(d2) -> Terminator11/1
  adc16x250-8/15(d3) -> Terminator12/1
  adc16x250-8/17(e1) -> sat4/1(In2)
  adc16x250-8/18(e2) -> Terminator13/1
  adc16x250-8/19(e3) -> Terminator14/1
  adc16x250-8/20(e4) -> Terminator15/1
  adc16x250-8/22(f2) -> Terminator17/1
  adc16x250-8/23(f3) -> Terminator18/1
  adc16x250-8/25(g1) -> sat6/1(In2)
  adc16x250-8/26(g2) -> Terminator19/1
  adc16x250-8/27(g3) -> Terminator20/1
  adc16x250-8/28(g4) -> Terminator21/1
  adc16x250-8/30(h2) -> Terminator23/1
  adc16x250-8/31(h3) -> Terminator24/1
  adc16x250-8/5(b1) -> sat1/1(In2)
  adc16x250-8/8(b4) -> Terminator5/1
  adc16x250-8/13(d1) -> sat3/1(In2)
  adc16x250-8/16(d4) -> Terminator10/1
  adc16x250-8/21(f1) -> sat5/1(In2)
  adc16x250-8/24(f4) -> Terminator16/1
  adc16x250-8/29(h1) -> sat7/1(In2)
  adc16x250-8/32(h4) -> Terminator22/1
